simulink model "MBD_FULL_VEHICLEMODEL"  (R2021b)
settings: Solver=VariableStepAuto  StartTime=0.0  StopTime=660  RelTol=1e-3
values from neighbouring files (symbols this model uses):
  rider_mass = 80    [MBD_Workspace_var.mat]
  tire_dia = 18    [MBD_Workspace_var.mat]
  vehicle_mass = 237    [MBD_Workspace_var.mat]
libraries: nesl_utility x26, fl_lib x24, sdl_lib x9, autolibshared x1, slpidlib x1
settings Model: Creator=vasan  LastModifiedBy=vasan

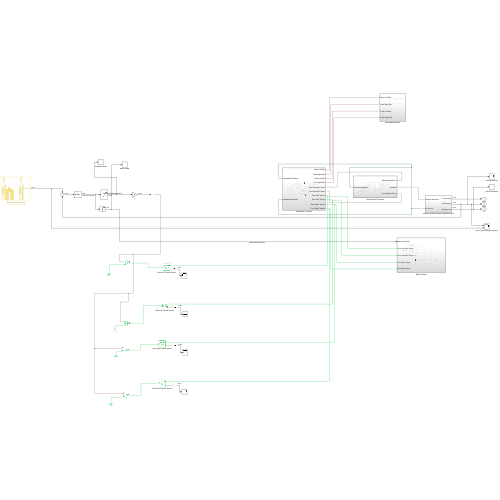
[thumbnail: Simulink's stored preview of the top-level diagram]
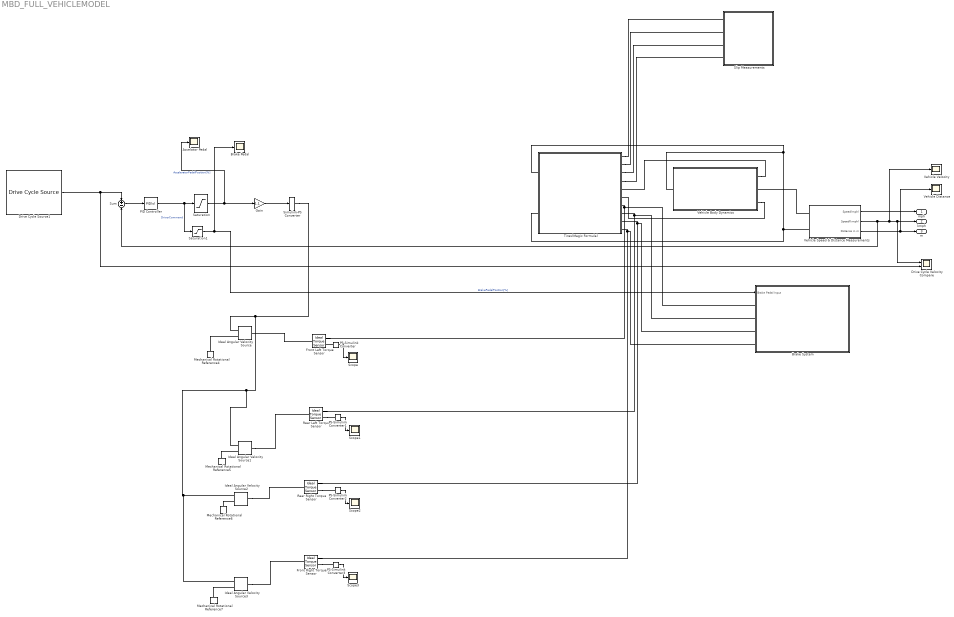
== system MBD_FULL_VEHICLEMODEL ==
  Accelator Pedal : Scope
  Brake Pedal : Scope
  Brake System : Subsystem
  Drive Cycle Source1 : autolibshared/Drive Cycle Source  cycleVar=FTP75  fileVar=cycleFTP75.mat  tfinal="2474  seconds"  cycleRepeat=off  outAccPort=off  outGearPort=off  gearList=No gear data  t_wot1=5  xdot_woto=0  xdot_wot1=30  t_wot2=20  xdot_wot2=0  t_wotend=30  srcUnit=m/s  outUnit=m/s  srcAccUnit=m/s/s  outAccUnit=m/s^2  dt=0  aMode=1  faultOption=off  velBnd=2  velBndUnit=mph  inUnit=m/s  timeBnd=1  failOption=off  stopSim=off  maxFaultCnt=10  maxFaultTime=2  maxTotFaultTime=15  traceOption=off  dtTrace=1  traceWindow=10  lastDCname=FTP75  lastOutUnit=mph  lastDT=0  lastTB=1  lastSB=2  forceCalcBound=off
      settings: SourceProductBaseCode=PW,DR,MT,UV,VE
  Drive Cycle Velocity Compare : Scope  NumInputPorts=2
  Front Left Torque Sensor : fl_lib/Mechanical/Mechanical Sensors/Ideal Torque Sensor
  Front Right Torque Sensor : fl_lib/Mechanical/Mechanical Sensors/Ideal Torque Sensor
  Gain : Gain  Gain=1.1
  Ideal Angular Velocity Source{,1..3} (4 alike) : fl_lib/Mechanical/Mechanical Sources/Ideal Angular Velocity Source
  Mechanical Rotational Reference{4..7} (4 alike) : fl_lib/Mechanical/Rotational Elements/Mechanical Rotational Reference
  PID Controller : slpidlib/PID Controller  Controller=PID  Form=Parallel  TimeDomain=Continuous-time  UseExternalTs=off  SampleTime=0.1  IntegratorMethod=Forward Euler  FilterMethod=Forward Euler  ControllerParametersSource=internal  P=7500  I=1  D=0  UseFilter=on  N=156169.602391718  TunerSelectOption=Transfer Function Based (PID Tuner App)  InitialConditionSource=internal  InitialConditionForIntegrator=0  InitialConditionForFilter=0  DifferentiatorICPrevScaledInput=0  ExternalReset=none  TrackingMode=off  Kt=1  LimitOutput=off  SatLimitsSource=internal  UpperSaturationLimit=inf  LowerSaturationLimit=-inf  LinearizeAsGain=on  AntiWindupMode=none  Kb=1  POutMin=[]  POutMax=[]  IOutMin=[]  IOutMax=[]  DOutMin=[]  DOutMax=[]  NOutMin=[]  NOutMax=[]  SumOutMin=[]  SumOutMax=[]  SaturationOutMin=[]  SaturationOutMax=[]  PParamMin=[]  PParamMax=[]  IParamMin=[]  IParamMax=[]  DParamMin=[]  DParamMax=[]  NParamMin=[]  NParamMax=[]  KbParamMin=[]  KbParamMax=[]  KtParamMin=[]  KtParamMax=[]  KbOutMin=[]  KbOutMax=[]  KtOutMin=[]  KtOutMax=[]  IntegratorOutMin=[]  IntegratorOutMax=[]  FilterOutMin=[]  FilterOutMax=[]  SumI1OutMin=[]  SumI1OutMax=[]  SumI2OutMin=[]  SumI2OutMax=[]  SumI3OutMin=[]  SumI3OutMax=[]  SumI4OutMin=[]  SumI4OutMax=[]  SumDOutMin=[]  SumDOutMax=[]  DifferentiatorOutMin=[]  DifferentiatorOutMax=[]  FilterDiffOutCoefMin=[]  FilterDiffOutCoefMax=[]  ReciprocalOutMin=[]  ReciprocalOutMax=[]  SumDenOutMin=[]  SumDenOutMax=[]  SumNumOutMin=[]  SumNumOutMax=[]  DivideOutMin=[]  DivideOutMax=[]  UdiffTsProdOutMin=[]  UdiffTsProdOutMax=[]  NTsProdOutMin=[]  NTsProdOutMax=[]  UintegralTsProdOutMin=[]  UintegralTsProdOutMax=[]  UngainTsProdOutMin=[]  UngainTsProdOutMax=[]  IntegratorContinuousStateAttributes=''  IntegratorStateMustResolveToSignalObject=off  IntegratorRTWStateStorageClass=Auto  FilterContinuousStateAttributes=''  FilterStateMustResolveToSignalObject=off  FilterRTWStateStorageClass=Auto  ParallelPVariant=InternalParameters  IdealPVariant=Disabled  IVariant=InternalParameters  DVariant=InternalParameters  IntegratorVariant=Continuous  SatVariant=Disabled  AWVariant=Passthrough  PCopyVariant=Disabled  TRVariant=Disabled  FdbkBlocksVariant=Forward  IdealPFdbkVariant=Disabled  SatFdbkVariant=Disabled  DerivativeFilterVariant=ContFilter  NVariant=InternalParameters  NCopyVariant=Disabled  FilterICVariant=InternalICsFilter  IntegratorICVariant=InternalICs  ExternalResetVariant=Disabled  TRSumVariant=Passthrough  SumFdbkVariant=Disabled  SumVariant=Sum_PID  TsampFilterVariant=InternalTs  TsampNgainVariant=Passthrough  TsampIntegralVariant=Passthrough  ExternalSaturationOutDataTypeStr=Inherit: Same as second input
  PS-Simulink Converter{,1..3} (4 alike) : nesl_utility/PS-Simulink Converter  PhysicalDomain=network_engine_domain  SubClassName=ps_output  LeftPortType=input  RightPortType=output  PseudoPeriodic=off  Frequencies=[]  Unit=N*m  AffineConversion=off
      settings: SourceProductBaseCode=PW,SS
  Rear Left Torque Sensor : fl_lib/Mechanical/Mechanical Sensors/Ideal Torque Sensor
  Rear Right Torque Sensor : fl_lib/Mechanical/Mechanical Sensors/Ideal Torque Sensor
  Saturation : Saturate  UpperLimit=100  LowerLimit=0  ZeroCross=off
  Saturation1 : Saturate  UpperLimit=100  LowerLimit=0  ZeroCross=off
  Scope{,1..3} (4 alike) : Scope
  Simulink-PS Converter : nesl_utility/Simulink-PS Converter  PhysicalDomain=network_engine_domain  SubClassName=ps_input  LeftPortType=input  RightPortType=output  PseudoPeriodic=off  Frequencies=[]  NoiseDistribution=none  NoiseParameters=[]  Unit=rad/s  AffineConversion=off  FilteringAndDerivatives=filter  SimscapeFilterOrder=1  InputFilterTimeConstant=0.001  UdotUserProvided=0
      settings: SourceProductBaseCode=PW,SS
  Slip Measurements : Subsystem
  Sum : Sum  Inputs=+-
  Tires(Magic Formula) : Subsystem
  Vehicle Body Dynamics : Subsystem
  Vehicle Distance : Scope
  Vehicle Speed & Distance Measurements : Subsystem
  Vehicle Velocity : Scope
  mph : Outport  VectorParamsAs1DForOutWhenUnconnected=off
  kmph : Outport  Port=2  VectorParamsAs1DForOutWhenUnconnected=off
  m : Outport  Port=3  VectorParamsAs1DForOutWhenUnconnected=off
  wires:
  Vehicle Speed & Distance Measurements/1(Speed(mph)) -> mph/1
  Vehicle Speed & Distance Measurements/2(Speed(kmph)) -> Sum/2, Drive Cycle Velocity Compare/1, kmph/1, Vehicle Velocity/1
  Vehicle Speed & Distance Measurements/3(Distance in m) -> m/1, Vehicle Distance/1
  Drive Cycle Source1/1 -> Drive Cycle Velocity Compare/2, Sum/1
  Sum/1 -> PID Controller/1
  Saturation1/1 -> Brake Pedal/1, Brake System/1(Brake Pedal Input)  "BrakePedalPosition[%]"
  Saturation/1 -> Accelator Pedal/1, Gain/1  "AcceleratorPedalPosition[%]"
  PID Controller/1 -> Saturation1/1, Saturation/1  "DriverCommand"
  PS-Simulink Converter/1 -> Scope/1
  PS-Simulink Converter1/1 -> Scope1/1
  PS-Simulink Converter2/1 -> Scope2/1
  PS-Simulink Converter3/1 -> Scope3/1
  Gain/1 -> Simulink-PS Converter/1
  connections:
  Vehicle Speed & Distance Measurements/LConn2 -- Tires(Magic Formula)/LConn1 -- Vehicle Body Dynamics/LConn1 -- Tires(Magic Formula)/LConn2
  Tires(Magic Formula)/RConn1 -- Slip Measurements/LConn1
  Tires(Magic Formula)/RConn2 -- Slip Measurements/LConn2
  Tires(Magic Formula)/RConn3 -- Slip Measurements/LConn3
  Tires(Magic Formula)/RConn4 -- Slip Measurements/LConn4
  Vehicle Body Dynamics/RConn1 -- Tires(Magic Formula)/RConn5
  Vehicle Speed & Distance Measurements/LConn1 -- Vehicle Body Dynamics/RConn2
  Vehicle Body Dynamics/RConn3 -- Tires(Magic Formula)/RConn6
  Brake System/LConn1 -- Front Left Torque Sensor/RConn1 -- Tires(Magic Formula)/RConn7
  Brake System/LConn2 -- Rear Left Torque Sensor/RConn1 -- Tires(Magic Formula)/RConn8
  Brake System/LConn3 -- Rear Right Torque Sensor/RConn1 -- Tires(Magic Formula)/RConn9
  Brake System/LConn4 -- Front Right Torque Sensor/RConn1 -- Tires(Magic Formula)/RConn10
  Simulink-PS Converter/RConn1 -- Ideal Angular Velocity Source/RConn1 -- Ideal Angular Velocity Source3/RConn1 -- Ideal Angular Velocity Source2/RConn1 -- Ideal Angular Velocity Source1/RConn1
  Ideal Angular Velocity Source/LConn1 -- Front Left Torque Sensor/LConn1
  Ideal Angular Velocity Source1/LConn1 -- Rear Left Torque Sensor/LConn1
  Ideal Angular Velocity Source2/LConn1 -- Rear Right Torque Sensor/LConn1
  Ideal Angular Velocity Source3/LConn1 -- Front Right Torque Sensor/LConn1
  PS-Simulink Converter/LConn1 -- Front Left Torque Sensor/RConn2
  Rear Left Torque Sensor/RConn2 -- PS-Simulink Converter1/LConn1
  Rear Right Torque Sensor/RConn2 -- PS-Simulink Converter2/LConn1
  Front Right Torque Sensor/RConn2 -- PS-Simulink Converter3/LConn1
  Mechanical Rotational Reference4/LConn1 -- Ideal Angular Velocity Source/RConn2
  Mechanical Rotational Reference5/LConn1 -- Ideal Angular Velocity Source1/RConn2
  Mechanical Rotational Reference6/LConn1 -- Ideal Angular Velocity Source2/RConn2
  Mechanical Rotational Reference7/LConn1 -- Ideal Angular Velocity Source3/RConn2

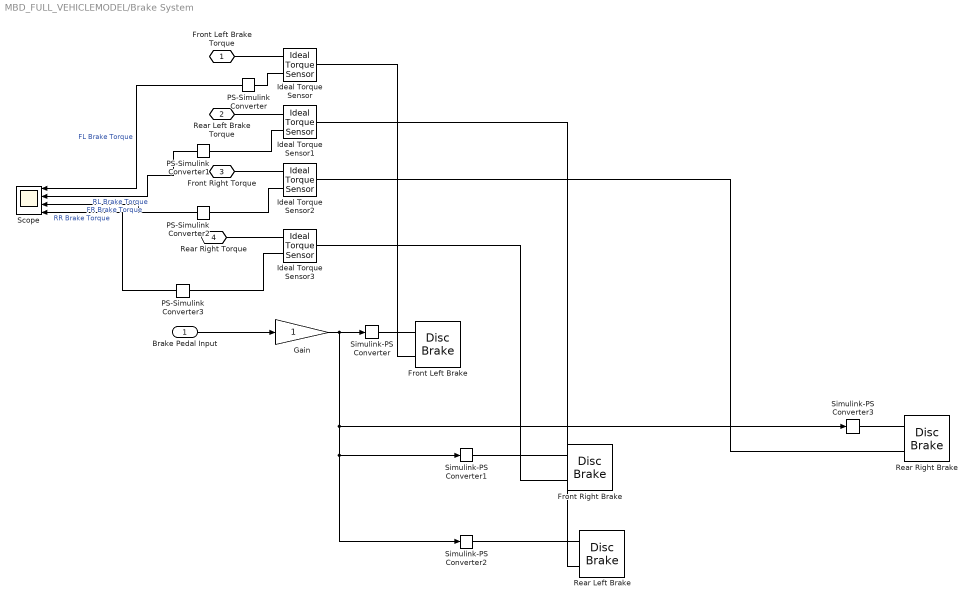
== system MBD_FULL_VEHICLEMODEL/Brake System ==
  Brake Pedal Input : Inport
  Front Left Brake : sdl_lib/Brakes & Detents/Rotational/Disc Brake  r_mean=150 mm  bore=10 mm  n_pads=2  thermal_port=simscape.enum.thermaleffects.omit  mu_static=0.9  mu_coulomb=0.7  temperature_TLU=[280, 300, 320] K  mu_static_TLU=[.9, .8, .7]  mu_coulomb_TLU=[.8, .7, .6]  brkwy_vel=0.1 rad/s  visc_coef=0 N*m*s/rad  enable_faults=simscape.enum.onoff.off  faulted_pressure=0 bar  external_fault=simscape.enum.onoff.off  temporal_fault=simscape.enum.onoff.off  fault_time=5 s  report_fault=simscape.enum.assert.action.none  thermal_mass=50 kJ/K  temperature_specify=off  temperature_priority=High  temperature=300 K  temperature_nominal_specify=off  temperature_nominal_unit=K  temperature_nominal_value=1
      settings: SourceProductBaseCode=LD
  Front Right Brake : sdl_lib/Brakes & Detents/Rotational/Disc Brake  r_mean=150 mm  bore=10 mm  n_pads=2  thermal_port=simscape.enum.thermaleffects.omit  mu_static=0.9  mu_coulomb=0.7  temperature_TLU=[280, 300, 320] K  mu_static_TLU=[.9, .8, .7]  mu_coulomb_TLU=[.8, .7, .6]  brkwy_vel=0.1 rad/s  visc_coef=0 N*m*s/rad  enable_faults=simscape.enum.onoff.off  faulted_pressure=0 bar  external_fault=simscape.enum.onoff.off  temporal_fault=simscape.enum.onoff.off  fault_time=5 s  report_fault=simscape.enum.assert.action.none  thermal_mass=50 kJ/K  temperature_specify=off  temperature_priority=High  temperature=300 K  temperature_nominal_specify=off  temperature_nominal_unit=K  temperature_nominal_value=1
      settings: SourceProductBaseCode=LD
  Gain : Gain
  Ideal Torque Sensor{,1..3} (4 alike) : fl_lib/Mechanical/Mechanical Sensors/Ideal Torque Sensor
  PS-Simulink Converter{,1..3} (4 alike) : nesl_utility/PS-Simulink Converter  PhysicalDomain=network_engine_domain  SubClassName=ps_output  LeftPortType=input  RightPortType=output  PseudoPeriodic=off  Frequencies=[]  Unit=inherit  AffineConversion=off
      settings: SourceProductBaseCode=PW,SS
  Rear Left Brake : sdl_lib/Brakes & Detents/Rotational/Disc Brake  r_mean=150 mm  bore=10 mm  n_pads=2  thermal_port=simscape.enum.thermaleffects.omit  mu_static=0.9  mu_coulomb=0.7  temperature_TLU=[280, 300, 320] K  mu_static_TLU=[.9, .8, .7]  mu_coulomb_TLU=[.8, .7, .6]  brkwy_vel=0.1 rad/s  visc_coef=0 N*m*s/rad  enable_faults=simscape.enum.onoff.off  faulted_pressure=0 bar  external_fault=simscape.enum.onoff.off  temporal_fault=simscape.enum.onoff.off  fault_time=5 s  report_fault=simscape.enum.assert.action.none  thermal_mass=50 kJ/K  temperature_specify=off  temperature_priority=High  temperature=300 K  temperature_nominal_specify=off  temperature_nominal_unit=K  temperature_nominal_value=1
      settings: SourceProductBaseCode=LD
  Rear Right Brake : sdl_lib/Brakes & Detents/Rotational/Disc Brake  r_mean=150 mm  bore=10 mm  n_pads=2  thermal_port=simscape.enum.thermaleffects.omit  mu_static=0.9  mu_coulomb=0.7  temperature_TLU=[280, 300, 320] K  mu_static_TLU=[.9, .8, .7]  mu_coulomb_TLU=[.8, .7, .6]  brkwy_vel=0.1 rad/s  visc_coef=0 N*m*s/rad  enable_faults=simscape.enum.onoff.off  faulted_pressure=0 bar  external_fault=simscape.enum.onoff.off  temporal_fault=simscape.enum.onoff.off  fault_time=5 s  report_fault=simscape.enum.assert.action.none  thermal_mass=50 kJ/K  temperature_specify=off  temperature_priority=High  temperature=300 K  temperature_nominal_specify=off  temperature_nominal_unit=K  temperature_nominal_value=1
      settings: SourceProductBaseCode=LD
  Scope : Scope  NumInputPorts=4
  Simulink-PS Converter{,1..3} (4 alike) : nesl_utility/Simulink-PS Converter  PhysicalDomain=network_engine_domain  SubClassName=ps_input  LeftPortType=input  RightPortType=output  PseudoPeriodic=off  Frequencies=[]  NoiseDistribution=none  NoiseParameters=[]  Unit=1  AffineConversion=off  FilteringAndDerivatives=provide  SimscapeFilterOrder=1  InputFilterTimeConstant=0.001  UdotUserProvided=0
      settings: SourceProductBaseCode=PW,SS
  Front Left Brake Torque : PMIOPort  Side=Left
  Rear Left Brake Torque : PMIOPort  Port=2  Side=Left
  Front Right Torque : PMIOPort  Port=3  Side=Left
  Rear Right Torque : PMIOPort  Port=4  Side=Left
  wires:
  Gain/1 -> Simulink-PS Converter3/1, Simulink-PS Converter2/1, Simulink-PS Converter1/1, Simulink-PS Converter/1
  Brake Pedal Input/1 -> Gain/1
  PS-Simulink Converter1/1 -> Scope/2  "RL Brake Torque"
  PS-Simulink Converter/1 -> Scope/1  "FL Brake Torque"
  PS-Simulink Converter2/1 -> Scope/3  "FR Brake Torque"
  PS-Simulink Converter3/1 -> Scope/4  "RR Brake Torque"
  connections:
  Simulink-PS Converter3/RConn1 -- Rear Right Brake/LConn1
  Simulink-PS Converter1/RConn1 -- Front Right Brake/LConn1
  Simulink-PS Converter/RConn1 -- Front Left Brake/LConn1
  Simulink-PS Converter2/RConn1 -- Rear Left Brake/LConn1
  Front Left Brake/LConn2 -- Ideal Torque Sensor/LConn1
  Ideal Torque Sensor/RConn1 -- Front Left Brake Torque/RConn1
  Ideal Torque Sensor1/LConn1 -- Rear Left Brake/LConn2
  Ideal Torque Sensor1/RConn1 -- Rear Left Brake Torque/RConn1
  Rear Right Brake/LConn2 -- Ideal Torque Sensor2/LConn1
  Front Right Torque/RConn1 -- Ideal Torque Sensor2/RConn1
  Front Right Brake/LConn2 -- Ideal Torque Sensor3/LConn1
  Ideal Torque Sensor3/RConn1 -- Rear Right Torque/RConn1
  PS-Simulink Converter/LConn1 -- Ideal Torque Sensor/RConn2
  PS-Simulink Converter1/LConn1 -- Ideal Torque Sensor1/RConn2
  PS-Simulink Converter2/LConn1 -- Ideal Torque Sensor2/RConn2
  PS-Simulink Converter3/LConn1 -- Ideal Torque Sensor3/RConn2

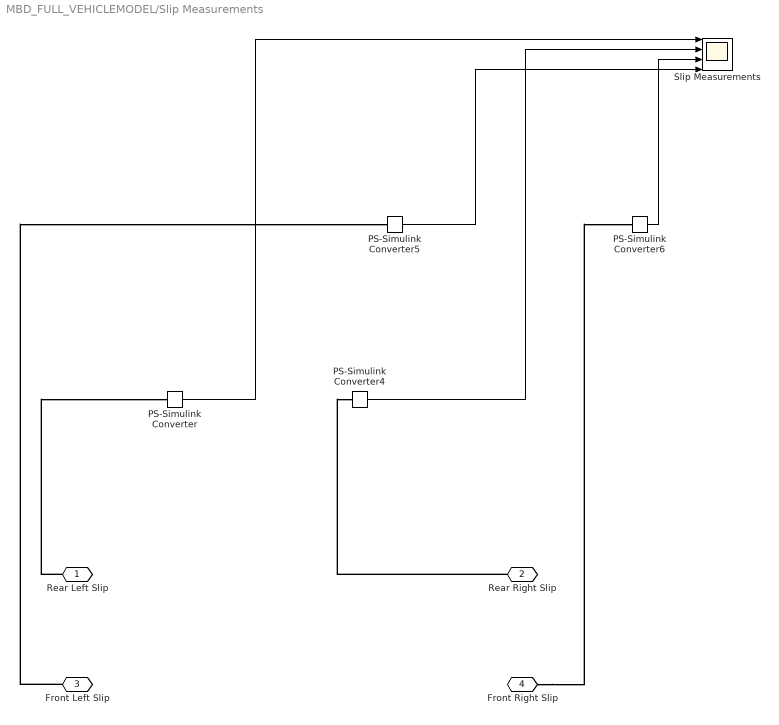
== system MBD_FULL_VEHICLEMODEL/Slip Measurements ==
  PS-Simulink Converter{,4..6} (4 alike) : nesl_utility/PS-Simulink Converter  PhysicalDomain=network_engine_domain  SubClassName=ps_output  LeftPortType=input  RightPortType=output  PseudoPeriodic=off  Frequencies=[]  Unit=inherit  AffineConversion=off
      settings: SourceProductBaseCode=PW,SS
  Slip Measurements : Scope  NumInputPorts=4
  Rear Left Slip : PMIOPort  Side=Left
  Rear Right Slip : PMIOPort  Port=2  Side=Left
  Front Left Slip : PMIOPort  Port=3  Side=Left
  Front Right Slip : PMIOPort  Port=4  Side=Left
  wires:
  PS-Simulink Converter4/1 -> Slip Measurements/2
  PS-Simulink Converter/1 -> Slip Measurements/1
  PS-Simulink Converter5/1 -> Slip Measurements/4
  PS-Simulink Converter6/1 -> Slip Measurements/3
  connections:
  Front Left Slip/RConn1 -- PS-Simulink Converter5/LConn1
  Rear Left Slip/RConn1 -- PS-Simulink Converter/LConn1
  Rear Right Slip/RConn1 -- PS-Simulink Converter4/LConn1
  Front Right Slip/RConn1 -- PS-Simulink Converter6/LConn1

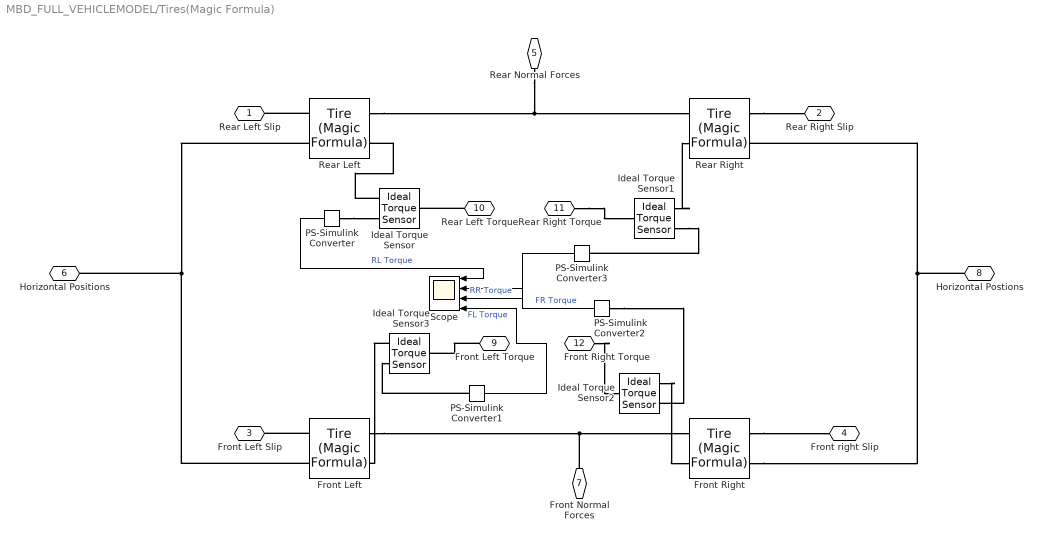
== system MBD_FULL_VEHICLEMODEL/Tires(Magic Formula) ==
  Front Left : sdl_lib/Tires & Vehicles/Tire (Magic Formula)  parameterization=sdl.enum.magic_tire_model.constant  F_z1=3000 N  F_x1=3500 N  kappa1=10  B_m=tire_b  C_m=tire_c  D_m=tire_d  E_m=tire_e  fz0=4000 N  p_Cx=1.685  p_Dx=[1.21, -.037]  p_Ex=[.344, .095, -.02, 0]  p_Kx=[21.51, -.163, .245]  p_Hx=[-.002, .002]  p_Vx=[0, 0]  r_e=tire_dia/2 in  model_compliance=sdl.enum.compliance.off  stiffness=1e6 N/m  damping=1000 N/(m/s)  model_inertia=sdl.enum.model_inertia.on  inertia=tire_inertia kg*m^2  initial_velocity=0 rad/s  model_resistance=simscape.enum.onoff.on  resistance_model=sdl.enum.rollingResistanceParameterization.constant  coeff=roll_resist  p_tire=250e3 Pa  alpha=-0.003  beta=0.97  coeff_a=84e-4  coeff_b=6.2e-4 s/m  coeff_c=1.6e-4 s^2/m^2  v_thr=0.001 m/s  v_tr_thr=0.1 m/s
  Front Right : sdl_lib/Tires & Vehicles/Tire (Magic Formula)  parameterization=sdl.enum.magic_tire_model.constant  F_z1=3000 N  F_x1=3500 N  kappa1=10  B_m=tire_b  C_m=tire_c  D_m=tire_d  E_m=tire_e  fz0=4000 N  p_Cx=1.685  p_Dx=[1.21, -.037]  p_Ex=[.344, .095, -.02, 0]  p_Kx=[21.51, -.163, .245]  p_Hx=[-.002, .002]  p_Vx=[0, 0]  r_e=tire_dia/2 in  model_compliance=sdl.enum.compliance.off  stiffness=1e6 N/m  damping=1000 N/(m/s)  model_inertia=sdl.enum.model_inertia.on  inertia=tire_inertia kg*m^2  initial_velocity=0 rad/s  model_resistance=simscape.enum.onoff.on  resistance_model=sdl.enum.rollingResistanceParameterization.constant  coeff=roll_resist  p_tire=250e3 Pa  alpha=-0.003  beta=0.97  coeff_a=84e-4  coeff_b=6.2e-4 s/m  coeff_c=1.6e-4 s^2/m^2  v_thr=0.001 m/s  v_tr_thr=0.1 m/s
  Ideal Torque Sensor{,1..3} (4 alike) : fl_lib/Mechanical/Mechanical Sensors/Ideal Torque Sensor
  PS-Simulink Converter{,1..3} (4 alike) : nesl_utility/PS-Simulink Converter  PhysicalDomain=network_engine_domain  SubClassName=ps_output  LeftPortType=input  RightPortType=output  PseudoPeriodic=off  Frequencies=[]  Unit=inherit  AffineConversion=off
      settings: SourceProductBaseCode=PW,SS
  Rear Left : sdl_lib/Tires & Vehicles/Tire (Magic Formula)  parameterization=sdl.enum.magic_tire_model.constant  F_z1=3000 N  F_x1=3500 N  kappa1=10  B_m=tire_b  C_m=tire_c  D_m=tire_d  E_m=tire_e  fz0=4000 N  p_Cx=1.685  p_Dx=[1.21, -.037]  p_Ex=[.344, .095, -.02, 0]  p_Kx=[21.51, -.163, .245]  p_Hx=[-.002, .002]  p_Vx=[0, 0]  r_e=tire_dia/2 in  model_compliance=sdl.enum.compliance.off  stiffness=1e6 N/m  damping=1000 N/(m/s)  model_inertia=sdl.enum.model_inertia.on  inertia=tire_inertia kg*m^2  initial_velocity=0 rad/s  model_resistance=simscape.enum.onoff.on  resistance_model=sdl.enum.rollingResistanceParameterization.constant  coeff=roll_resist  p_tire=250e3 Pa  alpha=-0.003  beta=0.97  coeff_a=84e-4  coeff_b=6.2e-4 s/m  coeff_c=1.6e-4 s^2/m^2  v_thr=0.001 m/s  v_tr_thr=0.1 m/s
  Rear Right : sdl_lib/Tires & Vehicles/Tire (Magic Formula)  parameterization=sdl.enum.magic_tire_model.constant  F_z1=3000 N  F_x1=3500 N  kappa1=10  B_m=tire_b  C_m=tire_c  D_m=tire_d  E_m=tire_e  fz0=4000 N  p_Cx=1.685  p_Dx=[1.21, -.037]  p_Ex=[.344, .095, -.02, 0]  p_Kx=[21.51, -.163, .245]  p_Hx=[-.002, .002]  p_Vx=[0, 0]  r_e=tire_dia/2 in  model_compliance=sdl.enum.compliance.off  stiffness=1e6 N/m  damping=1000 N/(m/s)  model_inertia=sdl.enum.model_inertia.on  inertia=tire_inertia kg*m^2  initial_velocity=0 rad/s  model_resistance=simscape.enum.onoff.on  resistance_model=sdl.enum.rollingResistanceParameterization.constant  coeff=roll_resist  p_tire=250e3 Pa  alpha=-0.003  beta=0.97  coeff_a=84e-4  coeff_b=6.2e-4 s/m  coeff_c=1.6e-4 s^2/m^2  v_thr=0.001 m/s  v_tr_thr=0.1 m/s
  Scope : Scope  NumInputPorts=4
  Rear Left Slip : PMIOPort  Side=Right
  Rear Right Slip : PMIOPort  Port=2  Side=Right
  Front Left Slip : PMIOPort  Port=3  Side=Right
  Front right Slip : PMIOPort  Port=4  Side=Right
  Rear Normal Forces : PMIOPort  Port=5  Side=Right
  Horizontal Positions : PMIOPort  Port=6  Side=Left
  Front Normal Forces : PMIOPort  Port=7  Side=Right
  Horizontal Postions : PMIOPort  Port=8  Side=Left
  Front Left Torque : PMIOPort  Port=9  Side=Right
  Rear Left Torque : PMIOPort  Port=10  Side=Right
  Rear Right Torque : PMIOPort  Port=11  Side=Right
  Front Right Torque : PMIOPort  Port=12  Side=Right
  wires:
  PS-Simulink Converter/1 -> Scope/1  "RL Torque"
  PS-Simulink Converter3/1 -> Scope/3  "RR Torque"
  PS-Simulink Converter2/1 -> Scope/2  "FR Torque"
  PS-Simulink Converter1/1 -> Scope/4  "FL Torque"
  connections:
  Front Left/LConn1 -- Front Normal Forces/RConn1 -- Front Right/LConn1
  Front Right/RConn2 -- Rear Right/RConn2 -- Horizontal Postions/RConn1
  Rear Left/RConn2 -- Front Left/RConn2 -- Horizontal Positions/RConn1
  Rear Left/LConn1 -- Rear Normal Forces/RConn1 -- Rear Right/LConn1
  Rear Left/RConn1 -- Rear Left Slip/RConn1
  Rear Right/RConn1 -- Rear Right Slip/RConn1
  Front Left/RConn1 -- Front Left Slip/RConn1
  Front Right/RConn1 -- Front right Slip/RConn1
  Rear Right Torque/RConn1 -- Ideal Torque Sensor1/LConn1
  Ideal Torque Sensor1/RConn1 -- Rear Right/LConn2
  Rear Left Torque/RConn1 -- Ideal Torque Sensor/LConn1
  Ideal Torque Sensor/RConn1 -- Rear Left/LConn2
  PS-Simulink Converter/LConn1 -- Ideal Torque Sensor/RConn2
  Ideal Torque Sensor1/RConn2 -- PS-Simulink Converter3/LConn1
  PS-Simulink Converter2/LConn1 -- Ideal Torque Sensor2/RConn2
  PS-Simulink Converter1/LConn1 -- Ideal Torque Sensor3/RConn2
  Front Right Torque/RConn1 -- Ideal Torque Sensor2/LConn1
  Ideal Torque Sensor2/RConn1 -- Front Right/LConn2
  Front Left Torque/RConn1 -- Ideal Torque Sensor3/LConn1
  Ideal Torque Sensor3/RConn1 -- Front Left/LConn2

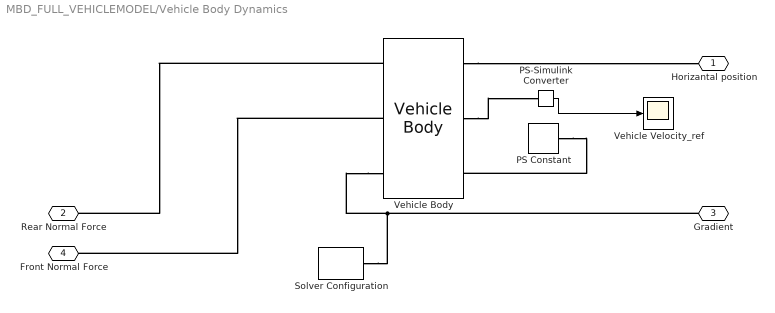
== system MBD_FULL_VEHICLEMODEL/Vehicle Body Dynamics ==
  PS Constant : fl_lib/Physical Signals/Sources/PS Constant  constant=0
  PS-Simulink Converter : nesl_utility/PS-Simulink Converter  PhysicalDomain=network_engine_domain  SubClassName=ps_output  LeftPortType=input  RightPortType=output  PseudoPeriodic=off  Frequencies=[]  Unit=inherit  AffineConversion=off
      settings: SourceProductBaseCode=PW,SS
  Solver Configuration : nesl_utility/Solver Configuration  PhysicalDomain=network_engine_domain  SubClassName=solver  LeftPortType=input  RightPortType=generic  Tones=[]  Harmonics=[]  SimulateNoise=off  Profile=off  UseLocalSampling=off  EnableSwitchedLinearOptims=on  FrequencyDomain=off  UseCCode=off  RelTol=0.001  AbsTol=1e-06  MinStep=1e-09  ToWorkspace=off  RevertToSquareIcSolve=off  NumHomotopyIterations=100  PhasorMode=off  PhasorModeNumHarmonics=1  DoDC=off  ResidualTolerance=1e-09  UseLocalSolver=off  LocalSolverChoice=NE_BACKWARD_EULER_ADVANCER  LocalSolverSampleTime=0.001  DoFixedCost=off  MaxNonlinIter=3  MaxModeIter=2  ComputeImpulses=off  ImpulseIterations=2  LinearAlgebra=auto  EquationFormulation=NE_TIME_EF  DelaysMemoryBudget=1024  AutomaticFiltering=on  FilteringTimeConstant=0.001  PartitionStorageMethod=AS_NEEDED  PartitionMemoryBudget=1024  PartitionMethod=ROBUST
      settings: SourceProductBaseCode=PW,SS
  Vehicle Body : sdl_lib/Tires & Vehicles/Vehicle Body  mass=rider_mass+vehicle_mass kg  n_w=2  x_f=front_axle_distance mm  x_r=rear_axle_distance mm  y_c=CG_height mm  mass_var=simscape.enum.onoff.off  g=9.81 m/s^2  liftoff_warning=simscape.enum.onoff.off  area=front_area m^2  Cd=drag_coeff  rho=1.18 kg/m^3  model_pitch=simscape.enum.onoff.off  inertia=4000 kg*m^2  suspension_model=sdl.enum.linearTLU.linear  k_f=1e4 N/m  b_f=1e4 N/(m/s)  k_r=1e4 N/m  b_r=1e4 N/(m/s)  k_f_TLU=[-2000, -1000, 0, 1000, 2000] N  x_f_TLU=[-.4, -.2, 0, .2, .4] m  b_f_TLU=[-200, -100, 0, 100, 200] N  v_f_TLU=[-4, -2, 0, 2, 4] m/s  k_r_TLU=[-2000, -1000, 0, 1000, 2000] N  x_r_TLU=[-.4, -.2, 0, .2, .4] m  b_r_TLU=[-200, -100, 0, 100, 200] N  v_r_TLU=[-4, -2, 0, 2, 4] m/s  interp_method=simscape.enum.interpolation.linear  extrap_method=simscape.enum.extrapolation.linear  model_hardstop=simscape.enum.onoff.off  upper_bound_f=.25 m  lower_bound_f=-.25 m  stop_k_f=1e6 N/m  stop_b_f=150 N/(m/s)  upper_bound_r=.25 m  lower_bound_r=-.25 m  stop_k_r=1e6 N/m  stop_b_r=150 N/(m/s)  initial_pitch=0 rad  initial_pitch_rate=0 rad/s  v_specify=on  v_priority=High  v=0 m/s  v_nominal_specify=off  v_nominal_unit=m/s  v_nominal_value=1
  Vehicle Velocity_ref : Scope
  Horizantal position : PMIOPort  Side=Left
  Rear Normal Force : PMIOPort  Port=2  Side=Right
  Gradient : PMIOPort  Port=3  Side=Right
  Front Normal Force : PMIOPort  Port=4  Side=Right
  wires:
  PS-Simulink Converter/1 -> Vehicle Velocity_ref/1
  connections:
  Vehicle Body/LConn1 -- Horizantal position/RConn1
  Vehicle Body/RConn1 -- Rear Normal Force/RConn1
  Vehicle Body/LConn2 -- PS-Simulink Converter/LConn1
  Vehicle Body/RConn2 -- Front Normal Force/RConn1
  Vehicle Body/RConn3 -- Gradient/RConn1 -- Solver Configuration/RConn1
  PS Constant/RConn1 -- Vehicle Body/LConn3

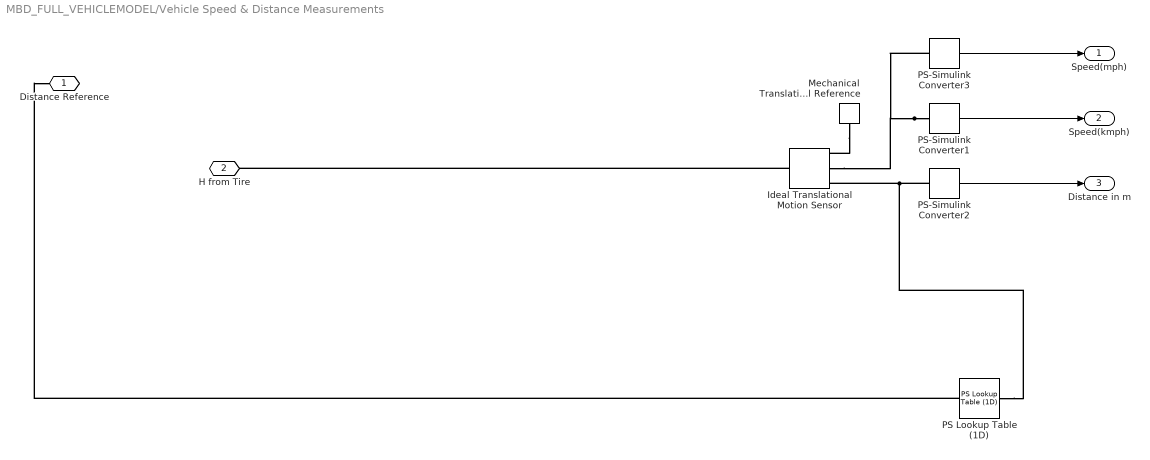
== system MBD_FULL_VEHICLEMODEL/Vehicle Speed & Distance Measurements ==
  Ideal Translational Motion Sensor : fl_lib/Mechanical/Mechanical Sensors/Ideal Translational Motion Sensor  offset=0 m
  Mechanical Translational Reference : fl_lib/Mechanical/Translational Elements/Mechanical Translational Reference
  PS Lookup Table (1D) : fl_lib/Physical Signals/Lookup Tables/PS Lookup Table (1D)  x=dist m  f=slope  interp_method=simscape.enum.interpolation.linear  extrap_method=simscape.enum.extrapolation.linear
      settings: SourceProductBaseCode=SS
  PS-Simulink Converter1 : nesl_utility/PS-Simulink Converter  PhysicalDomain=network_engine_domain  SubClassName=ps_output  LeftPortType=input  RightPortType=output  PseudoPeriodic=off  Frequencies=[]  Unit=km/hr  AffineConversion=off
  PS-Simulink Converter2 : nesl_utility/PS-Simulink Converter  PhysicalDomain=network_engine_domain  SubClassName=ps_output  LeftPortType=input  RightPortType=output  PseudoPeriodic=off  Frequencies=[]  Unit=inherit  AffineConversion=off
  PS-Simulink Converter3 : nesl_utility/PS-Simulink Converter  PhysicalDomain=network_engine_domain  SubClassName=ps_output  LeftPortType=input  RightPortType=output  PseudoPeriodic=off  Frequencies=[]  Unit=mph  AffineConversion=off
  Distance Reference : PMIOPort  Side=Left
  H from Tire : PMIOPort  Port=2  Side=Left
  Speed(mph) : Outport  VectorParamsAs1DForOutWhenUnconnected=off
  Speed(kmph) : Outport  Port=2  VectorParamsAs1DForOutWhenUnconnected=off
  Distance in m : Outport  Port=3  VectorParamsAs1DForOutWhenUnconnected=off
  wires:
  PS-Simulink Converter2/1 -> Distance in m/1
  PS-Simulink Converter1/1 -> Speed(kmph)/1
  PS-Simulink Converter3/1 -> Speed(mph)/1
  connections:
  PS-Simulink Converter1/LConn1 -- Ideal Translational Motion Sensor/RConn2 -- PS-Simulink Converter3/LConn1
  Mechanical Translational Reference/LConn1 -- Ideal Translational Motion Sensor/RConn1
  PS Lookup Table (1D)/RConn1 -- Distance Reference/RConn1
  PS-Simulink Converter2/LConn1 -- PS Lookup Table (1D)/LConn1 -- Ideal Translational Motion Sensor/RConn3
  Ideal Translational Motion Sensor/LConn1 -- H from Tire/RConn1
